simulink model "multi_Forword"  (R2021b)
settings: Solver=VariableStepAuto  StartTime=0.0  StopTime=0.013  RelTol=1e-3
libraries: spsSeriesRLCBranchLib x6, spsDiodeLib x5, spsCurrentMeasurementLib x3, spsVoltageMeasurementLib x3, spsLinearTransformerLib x2, spspowerguiLib x2, spsMosfetLib x1, spsDCVoltageSourceLib x1
settings Model: Creator=mouht  LastModifiedBy=mouht

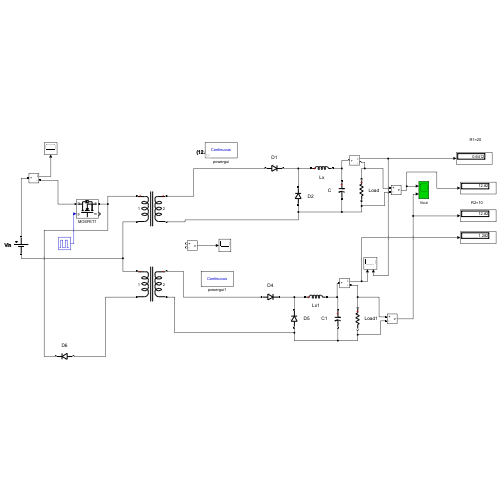
[thumbnail: Simulink's stored preview of the top-level diagram]
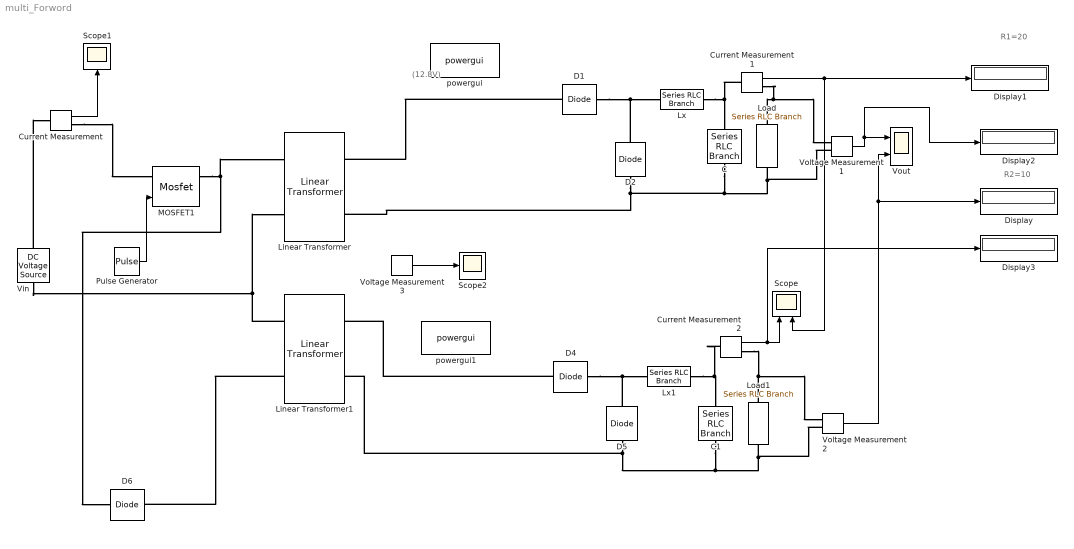
== system multi_Forword ==
  note: R2=10
  note: R1=20
  note: (12.8V)
  C : spsSeriesRLCBranchLib/Series RLC Branch  LConnTagsString=__new0  RConnTagsString=__new0  BranchType=C  Resistance=1e-4  Inductance=200e-6  SetiL0=off  InitialCurrent=0  Capacitance=100e-6  Setx0=off  InitialVoltage=0  Measurements=None
  C1 : spsSeriesRLCBranchLib/Series RLC Branch  LConnTagsString=__new0  RConnTagsString=__new0  BranchType=C  Resistance=1e-4  Inductance=200e-6  SetiL0=off  InitialCurrent=0  Capacitance=100e-6  Setx0=off  InitialVoltage=0  Measurements=None
  Current Measurement : spsCurrentMeasurementLib/Current Measurement  PhasorSimulation=off  OutputType=Complex  PSBequivalent=0
  Current Measurement1 : spsCurrentMeasurementLib/Current Measurement  PhasorSimulation=off  OutputType=Complex  PSBequivalent=0
  Current Measurement2 : spsCurrentMeasurementLib/Current Measurement  PhasorSimulation=off  OutputType=Complex  PSBequivalent=0
  D{1..2,4..6} (5 alike) : spsDiodeLib/Diode  Ron=1e-3  Lon=0  Vf=0  IC=0  UseSnubber=off  Rs=inf  Cs=0  Measurements=off
  Display{,1..3} (4 alike) : Display
  Linear Transformer : spsLinearTransformerLib/Linear Transformer  UNITS=SI  NominalPower=[ 25 100e3 ]  winding1=[48 0 0]  winding2=[32 0 0]  ThreeWindings=off  winding3=[48 0 0]  RmLm=[inf 10e-3]  Measurements=Magnetization current  DataType=on
  Linear Transformer1 : spsLinearTransformerLib/Linear Transformer  UNITS=SI  NominalPower=[ 25 100e3 ]  winding1=[48 0 0]  winding2=[32 0 0]  ThreeWindings=off  winding3=[48 0 0]  RmLm=[inf 10e-3]  Measurements=Magnetization current  DataType=on
  Load : spsSeriesRLCBranchLib/Series RLC Branch  LConnTagsString=__new0  RConnTagsString=__new0  BranchType=R  Resistance=20  Inductance=200e-6  SetiL0=off  InitialCurrent=0  Capacitance=400e-6  Setx0=off  InitialVoltage=0  Measurements=Branch current
  Load1 : spsSeriesRLCBranchLib/Series RLC Branch  LConnTagsString=__new0  RConnTagsString=__new0  BranchType=R  Resistance=10  Inductance=200e-6  SetiL0=off  InitialCurrent=0  Capacitance=400e-6  Setx0=off  InitialVoltage=0  Measurements=Branch current
  Lx : spsSeriesRLCBranchLib/Series RLC Branch  LConnTagsString=__new0  RConnTagsString=__new0  BranchType=L  Resistance=10  Inductance=400e-6  SetiL0=off  InitialCurrent=0  Capacitance=400e-6  Setx0=off  InitialVoltage=0  Measurements=Branch current
  Lx1 : spsSeriesRLCBranchLib/Series RLC Branch  LConnTagsString=__new0  RConnTagsString=__new0  BranchType=L  Resistance=10  Inductance=400e-6  SetiL0=off  InitialCurrent=0  Capacitance=400e-6  Setx0=off  InitialVoltage=0  Measurements=Branch current
  MOSFET1 : spsMosfetLib/Mosfet  Ron=1e-6  Lon=0  Rd=1e-6  Vfd=0  IC=0  Rs=1e6  Cs=inf  Measurements=on
  Pulse Generator : DiscretePulseGenerator  PulseType=Time based  Period=1/35e3  PulseWidth=40
  Scope : Scope  NumInputPorts=2
  Scope1 : Scope
  Scope2 : Scope
  Vin : spsDCVoltageSourceLib/DC Voltage Source  Amplitude=48  Measurements=None
  Voltage Measurement1 : spsVoltageMeasurementLib/Voltage Measurement  PhasorSimulation=off  OutputType=Complex  PSBequivalent=0
  Voltage Measurement2 : spsVoltageMeasurementLib/Voltage Measurement  PhasorSimulation=off  OutputType=Complex  PSBequivalent=0
  Voltage Measurement3 : spsVoltageMeasurementLib/Voltage Measurement  PhasorSimulation=off  OutputType=Complex  PSBequivalent=0
  Vout : Scope  NumInputPorts=2
  powergui : spspowerguiLib/powergui  Priority=1  SimulationMode=Continuous  SampleTime=50e-6  frequency=60  Iterations=50  frequencyindice=0  Pbase=100e6  ErrMax=1e-4  UnitsV=kV  UnitsW=MW  buscounter=0  FunctionMessages=off  echomessages=off  EnableUseOfTLC=off  CurrentSourceSwitches=off  DisableSnubberDevices=off  DisableRonSwitches=off  DisableVfSwitches=off  DisplayEquations=off  AutomaticDiscreteSolvers=off  SolverType=Tustin/Backward Euler (TBE)  Interpol=off  ExternalGateDelay=off  methode=off  Ts=100  x0status=blocks  SPID=on  SwTol=0  HookPort=off  NonlinearTolerance=1e-4  nMaxIteration=100  ContinueOnMaxIteration=off  RestoreLinks=warning  ResistiveCurrentMeasurement=off  Frange=[0:2:500]  Ylog=off  Xlog=on  ShowGrid=off  save=off  variable=ZData  structure=0  ZoomFFT=off  StartTime=0.0  cycles=1  DisplayStyle=1  fundamental=60  FreqAxis=off  MaxFrequency=1000  frequencyindicesteady=1  RmsSteady=1  display=off
  powergui1 : spspowerguiLib/powergui  Priority=1  SimulationMode=Continuous  SampleTime=50e-6  frequency=60  Iterations=50  frequencyindice=0  Pbase=100e6  ErrMax=1e-4  UnitsV=kV  UnitsW=MW  buscounter=0  FunctionMessages=off  echomessages=off  EnableUseOfTLC=off  CurrentSourceSwitches=off  DisableSnubberDevices=off  DisableRonSwitches=off  DisableVfSwitches=off  DisplayEquations=off  AutomaticDiscreteSolvers=off  SolverType=Tustin/Backward Euler (TBE)  Interpol=off  ExternalGateDelay=off  methode=off  Ts=100  x0status=blocks  SPID=on  SwTol=0  HookPort=off  NonlinearTolerance=1e-4  nMaxIteration=100  ContinueOnMaxIteration=off  RestoreLinks=warning  ResistiveCurrentMeasurement=off  Frange=[0:2:500]  Ylog=off  Xlog=on  ShowGrid=off  save=off  variable=ZData  structure=0  ZoomFFT=off  StartTime=0.0  cycles=1  DisplayStyle=1  fundamental=60  FreqAxis=off  MaxFrequency=1000  frequencyindicesteady=1  RmsSteady=1  display=off
  wires:
  Current Measurement/1 -> Scope1/1
  Voltage Measurement1/1 -> Display2/1, Vout/1
  Voltage Measurement2/1 -> Vout/2, Display/1
  Current Measurement1/1 -> Scope/2, Display1/1
  Current Measurement2/1 -> Display3/1, Scope/1
  Voltage Measurement3/1 -> Scope2/1
  Pulse Generator/1 -> MOSFET1/1
  connections:
  Load/LConn1 -- Current Measurement1/RConn1 -- Voltage Measurement1/LConn1
  Load/RConn1 -- Voltage Measurement1/LConn2 -- D2/LConn1 -- Linear Transformer/RConn2 -- C/RConn1
  D1/RConn1 -- D2/RConn1 -- Lx/LConn1
  Vin/RConn1 -- Current Measurement/LConn1
  D1/LConn1 -- Linear Transformer/RConn1
  Lx1/RConn1 -- Current Measurement2/LConn1 -- C1/LConn1
  Load1/RConn1 -- Voltage Measurement2/LConn2 -- D5/LConn1 -- Linear Transformer1/RConn2 -- C1/RConn1
  D4/RConn1 -- D5/RConn1 -- Lx1/LConn1
  D4/LConn1 -- Linear Transformer1/RConn1
  Linear Transformer1/LConn1 -- Vin/LConn1 -- Linear Transformer/LConn2
  Lx/RConn1 -- Current Measurement1/LConn1 -- C/LConn1
  Load1/LConn1 -- Current Measurement2/RConn1 -- Voltage Measurement2/LConn1
  MOSFET1/RConn1 -- Linear Transformer/LConn1 -- D6/RConn1
  Current Measurement/RConn1 -- MOSFET1/LConn1
  Linear Transformer1/LConn2 -- D6/LConn1
